simulink model "sns_units_spk_hybrid"  (R2025a)
settings: Solver=ode45  StartTime=0.0  StopTime=0.5  RelTol=1e-8  AbsTol=1e-10
libraries: SNS_Library x3
settings Model: Creator=Ben Bolen  LastModifiedBy=Ben Bolen
settings DataIOCC: SignalLoggingName=sigs

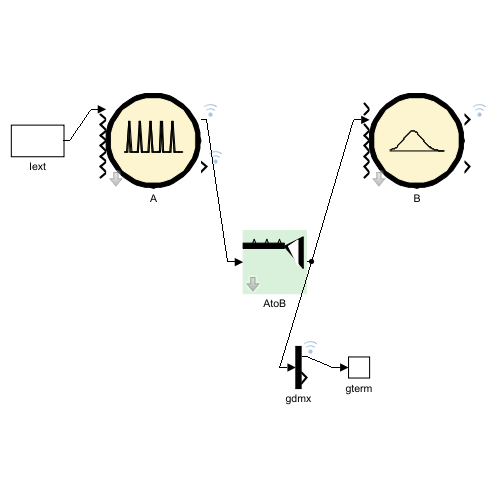
[thumbnail: Simulink's stored preview of the top-level diagram]
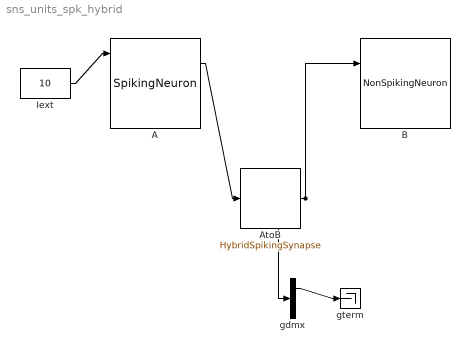
== system sns_units_spk_hybrid ==
  A : SNS_Library/SpikingNeuron  Vrest=0  Vth=8  Vreset=0  Gm=1  Cm=5
  AtoB : SNS_Library/HybridSpikingSynapse  gmax=0.3  ginc=0.1  tau_syn=100  Esyn=8  ThrPre=7.5
  B : SNS_Library/NonSpikingNeuron  Vrest=0  Gm=1  Cm=200  Thr=0  Slope=5
  Iext : Constant  Value=10
  gdmx : Demux  Outputs=2
  gterm : Terminator
  wires:
  Iext/1 -> A/1
  A/1 -> AtoB/1
  AtoB/1 -> B/2, gdmx/1
  gdmx/1 -> gterm/1
